simulink model "quadcopter_sim"  (Simulink 7.7)
settings: Solver=ode45  StartTime=0.0  StopTime=500000  RelTol=1e-3
undefined symbols (not defined in the file or in its folder): fuzzy_system, fuzzy_system_yaw, quadcopter
libraries: simulink x2
settings Model: Creator=Diego  LastModifiedBy=Diego

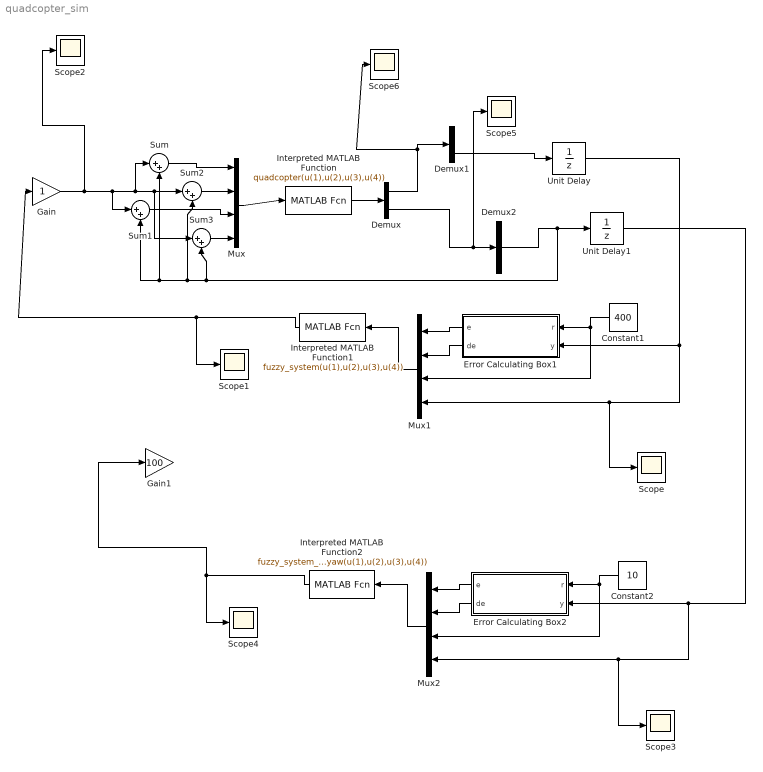
== system quadcopter_sim ==
  Constant1 : Constant  Value=400  SampleTime=10
  Constant2 : Constant  Value=10  SampleTime=10
  Demux : Demux  Outputs=2
  Demux1 : Demux  Outputs=3
  Demux2 : Demux  Outputs=3
  Error Calculating Box1 : Subsystem
  Error Calculating Box2 : Subsystem
  Gain : Gain
  Gain1 : Gain  Gain=100
  Interpreted MATLAB Function : MATLABFcn  MATLABFcn=quadcopter(u(1),u(2),u(3),u(4))  Output1D=off
  Interpreted MATLAB Function1 : MATLABFcn  MATLABFcn=fuzzy_system(u(1),u(2),u(3),u(4))  SampleTime=1
  Interpreted MATLAB Function2 : MATLABFcn  MATLABFcn=fuzzy_system_yaw(u(1),u(2),u(3),u(4))
  Mux : Mux
  Mux1 : Mux
  Mux2 : Mux
  Scope{,1..6} (7 alike) : Scope
      Scope settings: TimeRange=500000  YMin=0  YMax=600
      Scope1 settings: YMin=-750000  YMax=1.5e+006
      Scope2 settings: TimeRange=500000  YMin=-1.75e+006  YMax=1.75e+006  SaveName=ScopeData2
      Scope3 settings: YMin=-0.0004  YMax=0.0004  SaveName=ScopeData3
      Scope4 settings: YMin=2700  YMax=2950  SaveName=ScopeData4
      Scope5 settings: TimeRange=500000  YMin=0  SaveName=ScopeData5
      Scope6 settings: YMin=-50  YMax=450  SaveName=ScopeData6
  Sum{,1..3} (4 alike) : Sum  Inputs=|++
  Unit Delay : UnitDelay  SampleTime=-1
  Unit Delay1 : UnitDelay  SampleTime=-1
  wires:
  Mux/1 -> Interpreted MATLAB Function/1
  Interpreted MATLAB Function/1 -> Demux/1
  Constant1/1 -> Error Calculating Box1/1(r), Mux1/3
  Error Calculating Box1/1(e) -> Mux1/1
  Error Calculating Box1/2(de) -> Mux1/2
  Mux1/1 -> Interpreted MATLAB Function1/1
  Interpreted MATLAB Function1/1 -> Scope1/1, Gain/1
  Gain/1 -> Scope2/1, Sum1/1, Sum/1, Sum2/1, Sum3/1
  Demux/1 -> Demux1/1, Scope6/1
  Demux1/3 -> Unit Delay/1
  Unit Delay/1 -> Error Calculating Box1/2(y), Mux1/4, Scope/1
  Constant2/1 -> Error Calculating Box2/1(r), Mux2/3
  Error Calculating Box2/1(e) -> Mux2/1
  Error Calculating Box2/2(de) -> Mux2/2
  Mux2/1 -> Interpreted MATLAB Function2/1
  Interpreted MATLAB Function2/1 -> Scope4/1, Gain1/1
  Demux/2 -> Demux2/1, Scope5/1
  Sum/1 -> Mux/1
  Sum1/1 -> Mux/3
  Sum2/1 -> Mux/2
  Sum3/1 -> Mux/4
  Unit Delay1/1 -> Error Calculating Box2/2(y), Mux2/4, Scope3/1
  Demux2/2 -> Unit Delay1/1, Sum3/2, Sum2/2, Sum1/2, Sum/2

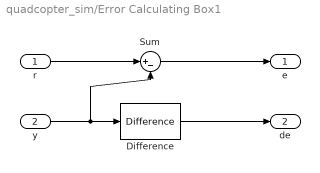
== system quadcopter_sim/Error Calculating Box1 ==
  r : Inport
  y : Inport  Port=2
  Difference : simulink/Discrete/Difference  SystemSampleTime=-1  ICPrevInput=0.0  OutMin=[]  OutMax=[]  OutDataType=fixdt(1, 16)  OutScaling=2^-10  DoSatur=off
  Sum : Sum  Inputs=|+-  SampleTime=1
  e : Outport
  de : Outport  Port=2
  wires:
  y/1 -> Difference/1, Sum/2
  Difference/1 -> de/1
  Sum/1 -> e/1
  r/1 -> Sum/1

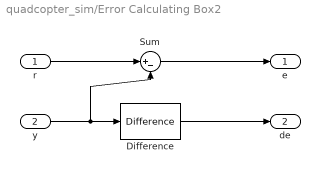
== system quadcopter_sim/Error Calculating Box2 ==
  r : Inport
  y : Inport  Port=2
  Difference : simulink/Discrete/Difference  SystemSampleTime=-1  ICPrevInput=0.0  OutMin=[]  OutMax=[]  OutDataType=fixdt(1, 16)  OutScaling=2^-10  DoSatur=off
  Sum : Sum  Inputs=|+-  SampleTime=1
  e : Outport
  de : Outport  Port=2
  wires:
  y/1 -> Difference/1, Sum/2
  Difference/1 -> de/1
  Sum/1 -> e/1
  r/1 -> Sum/1
